simulink model "battery_system_CV_PID"  (R2022a)
settings: Solver=VariableStepAuto  StartTime=0.0  StopTime=10.0  RelTol=1e-3
model workspace (MAT data in the model file):
  AN.EqPotentialHandle = 'E_eqGraphite'
  AN.i_oHandle = 'i_oC6'
  AN.sigmaHandle = 'sigmaC6'
  AN.D_oHandle = 'D_o_Graphite'
  AN.k_o = 3.80589129595e-09
  AN.alpha_a = 0.5
  AN.alpha_c = 0.5
  AN.C_dl = 3e-06
  AN.R_SEI = 0.00733702042142
  AN.sigma = 100
  AN.D_o = 3e-13
  AN.MW = 72.0642
  AN.MW_Lith = 79.0052
  AN.specCap = 350
  AN.rho = 2266
  AN.c_p = 720
  AN.k = 0.6
  AN.C_Li_max = 28.4851292094
  AN.del_z = 0.316227766017
  AN.del_y = 0.316227766017
  AN.L = 0.0001
  AN.r_p = 1.25e-05
  AN.eps_ed = 0.320700992698
  AN.eps_b = 0.172
  AN.A_geo = 1
  AN.gamma_brug = 1
  AN.alpha_brug = 1.5
  AN.del_x = 1e-05
  AN.x_vec = [5e-06 1.5e-05 2.5e-05 3.5e-05 4.5e-05 5.5e-05 6.5e-05 7.5e-05 8.5e-05 9.5e-05]
  AN.x_half_vec = [0 1e-05 2e-05 3e-05 4e-05 5e-05 6e-05 7e-05 8e-05 9e-05 0.0001]
  AN.del_r = 1.25e-06
  AN.r_vec = [6.25e-07 1.875e-06 3.125e-06 4.375e-06 5.625e-06 6.875e-06 8.125e-06 9.375e-06 1.0625e-05 1.1875e-05]
  AN.r_half_vec = [0 1.25e-06 2.5e-06 3.75e-06 5e-06 6.25e-06 7.5e-06 8.75e-06 1e-05 1.125e-05 1.25e-05]
  AN.eps_el = 0.507299007302
  AN.A_c = 0.1
  AN.Vol = 1e-05
  AN.dVol = 1e-06
  AN.V_sphere = 8.18123086872e-15
  AN.V_ed = 3.20700992698e-06
  AN.V_el = 5.07299007302e-06
  AN.dVol_el = 5.07299007302e-07
  AN.Np_tot = 391996018.501
  AN.Np_CV = 39199601.8501
  AN.A_surf = 1.96349540849e-09
  AN.A_surf_tot = 0.769682382475
  AN.A_surf_CV = 0.0769682382475
  AN.A_s = 76968.2382475
  AN.dVol_r = [8.18123086872e-18; 5.72686160811e-17; 1.55443386506e-16; 3.02705542143e-16; 4.99055082992e-16; 7.44492009054e-16; 1.03901632033e-15; 1.38262801681e-15; 1.77532709851e-15; 2.21711356542e-15]
  AN.Cap = 2.44837153197
  C = [0 0 -0.999999993923 0 0 0 0 0 0 0 0 0 0 0 0 0 0 0 0 0 0 0 0 0 0 0 0 0 0 0 0 0 0 0 0 0 0 0 0 0 0 0 0 0 0 0 0 0 0 0 0 0 0 0 0 0 0 0 0 0 0 0 0 0 0 0 0 0 0 0 0 0 0 0 0 0 0 0 0 0 0 0 0 0 0 0 0 0 0 0 0 0 0 0 0 0 0 0 0 0 0 0 0 0 0 0 0 0 0 0 0 0 0 0 0 0 0 0 0 0 0 0 0 0 0 0 0 0 0 0 0 0 0 0 0 0 0 0 0 0 0 0 0 0 0 0 0 0 0 0 0 0 0 0 0 0 0 0 0 0 0 0 0 0 0 0 0 0 0 0 0 0 0 0 0 0 0 0 0 0 0 0 0 0 0 0 0 0 0 0 0 0 0 0 0 0 0 0 0 0 0 0 0 0 0 0 0 0 0 0 0 0 0 0 0 0 0 0 0 0 0 0 0 0 0 0 0 0 0 0 0 0 0 0 0 0 0 0 0 0 0 0 0 0 0 0 0 0 0 0 0 0 0 0 0 0 0 0 0 0 0 0 0 0 0 0 0 0 0 0 0 0 0 0 0 0 0 0 0 0 0 0 0 0 0 0 0 0 0 0 0 0 0 0 0 0 0 0 0 0 0 0 0 0 0 0 0 0 0 0 0 0 0 0 0 0 0 0 0 0 0 0 0 0 0 0 0 0 0 0 0 0 0 0 0 0 0 0 0 0 0.999999999995 0 0 0 0 0 0 0 0 0 0 0 0 0 0]
  CA.EqPotentialHandle = 'E_eqNMC'
  CA.i_oHandle = 'i_oC6'
  CA.sigmaHandle = 'sigmaNMC'
  CA.D_oHandle = 'D_o_NMC532'
  CA.k_o = 9.72997022034e-10
  CA.alpha_a = 0.5
  CA.alpha_c = 0.5
  CA.C_dl = 1e-06
  CA.R_SEI = 0.00611911635272
  CA.sigma = 3.8
  CA.D_o = 5e-13
  CA.MW = 89.61275
  CA.MW_Lith = 96.55375
  CA.specCap = 170
  CA.rho = 2739.6961
  CA.c_p = 720
  CA.k = 0.6
  CA.C_Li_max = 40.5441490868
  CA.del_z = 0.316227766017
  CA.del_y = 0.316227766017
  CA.L = 0.0001
  CA.r_p = 5e-06
  CA.eps_ed = 0.442994582877
  CA.eps_b = 0.259
  CA.A_geo = 1
  CA.gamma_brug = 1
  CA.alpha_brug = 1.5
  CA.del_x = 1e-05
  CA.x_vec = [0.000135 0.000145 0.000155 0.000165 0.000175 0.000185 0.000195 0.000205 0.000215 0.000225]
  CA.x_half_vec = [0.00013 0.00014 0.00015 0.00016 0.00017 0.00018 0.00019 0.0002 0.00021 0.00022 0.00023]
  CA.del_r = 5e-07
  CA.r_vec = [2.5e-07 7.5e-07 1.25e-06 1.75e-06 2.25e-06 2.75e-06 3.25e-06 3.75e-06 4.25e-06 4.75e-06]
  CA.r_half_vec = [0 5e-07 1e-06 1.5e-06 2e-06 2.5e-06 3e-06 3.5e-06 4e-06 4.5e-06 5e-06]
  CA.eps_el = 0.298005417123
  CA.A_c = 0.1
  CA.Vol = 1e-05
  CA.dVol = 1e-06
  CA.V_sphere = 5.23598775598e-16
  CA.V_ed = 4.42994582877e-06
  CA.V_el = 2.98005417123e-06
  CA.dVol_el = 2.98005417123e-07
  CA.Np_tot = 8460573315.33
  CA.Np_CV = 846057331.533
  CA.A_surf = 3.14159265359e-10
  CA.A_surf_tot = 2.65796749726
  CA.A_surf_CV = 0.265796749726
  CA.A_s = 265796.749726
  CA.dVol_r = [5.23598775598e-19; 3.66519142919e-18; 9.94837673637e-18; 1.93731546971e-17; 3.19395253115e-17; 4.76474885794e-17; 6.6497044501e-17; 8.84881930761e-17; 1.13620934305e-16; 1.41895268187e-16]
  CA.Cap = 4.81377102891
  CONS.F = 96485338.3
  CONS.R = 8314.472
  CONS.T = 298.15
  CV_ref = 3.74905480499
  EL.tf_numHandle = 'transferenceNumber'
  EL.ActivityHandle = 'activity'
  EL.D_o_Li_ionHandle = 'D_oLiion'
  EL.kappaHandle = 'kappa'
  EL.D_o_Li_ion = 7.5e-11
  EL.kappa = 0.28
  EL.C = 1
  EL.tf_num = 0.363
  EL.Activity = 1
  EL.rho = 2266
  EL.c_p = 720
  EL.k = 470
  EL.gamma_brug = 1
  EL.alpha_brug = 1.5
  FLAG.AN_LI_FOIL = 0
  FLAG.CA_LI_FOIL = 0
  FLAG.R_AN = 1
  FLAG.R_CA = 1
  FLAG.COE = 0
  FLAG.T_BC_AN = 4
  FLAG.T_BC_CA = 4
  FLAG.CV_CONV = 0
  FLAG.HEAT_GEN_TOTAL = 1
  FLAG.HEAT_GEN_IONIC = 1
  FLAG.HEAT_GEN_ELECTRIC = 1
  FLAG.HEAT_GEN_RXN = 1
  FLAG.HEAT_GEN_CHEM_RXN = 0
  FLAG.V_SEI = 1
  FLAG.SEI_growth = 0
  FLAG.HeatGen = 0
  FLAG.Bruggeman = 0
  FLAG.BRUG_ED = 1
  FLAG.BRUG_EL = 1
  FLAG.BRUG_sigma = 1
  FLAG.BRUG_kappa = 1
  FLAG.BRUG_activity = 0
  FLAG.BRUG_D_Liion = 1
  FLAG.BRUG_tf_num = 0
  FLAG.BRUG_D_o_AN = 0
  FLAG.BRUG_D_o_CA = 0
  FLAG.Newman_i_o = 1
  FLAG.preDefined_C_max = 1
  FLAG.CONSTANT_PROPS_FROM_HANDLES = 0
  FLAG.VARIABLE_PROPS_FROM_HANDLES = 0
  FLAG.VARIABLE_kappa = 1
  FLAG.VARIABLE_activity = 0
  FLAG.VARIABLE_D_Liion = 0
  FLAG.VARIABLE_tf_num = 0
  FLAG.VARIABLE_D_o_AN = 0
  FLAG.VARIABLE_D_o_CA = 0
  FLAG.SaveSolnDiscreteTime = 1
  FLAG.SaveSystemForEst = 0
  FLAG.doPostProcessing = 1
  FLAG.ReduceSolnTime = 0
  FLAG.Plot = 1
  FLAG.PRBS_predefinded = 0
  K_D = 0
  K_I = -7437.93380511
  K_P = 0
  K_algb = [0 0 0 0 0 0 0 0 0 0 0 0 ... (126025 elements, 355x355)]
  M_cross = [1 0 0 0 0 0 0 0 0 0 0 0 ... (126025 elements, 355x355)]
  N.N_CV_AN = 10
  N.N_CV_SEP = 5
  N.N_CV_CA = 10
  N.N_R_AN = 10
  N.N_R_CA = 10
  N.N_R_max = 10
  N.N_ES_var = 6
  N.N_SV_nR = 7
  N.N_SV_SEP = 3
  N.N_prop = 19
  N.N_SV_AN = 17
  N.N_SV_CA = 17
  N.N_SV_AN_tot = 170
  N.N_SV_SEP_tot = 15
  N.N_SV_CA_tot = 170
  N.N_SV_tot = 355
  N.N_CV_tot = 25
  N.CV_Region_AN = [1 2 3 4 5 6 7 8 9 10]
  N.CV_Region_SEP = [11 12 13 14 15]
  N.CV_Region_CA = [16 17 18 19 20 21 22 23 24 25]
  N.N_diff = 270
  N.N_algb = 85
  P.T = 1
  P.del_phi = 2
  P.phi_ed = 3
  P.V_1 = 4
  P.V_2 = 5
  P.i_PS = 6
  P.C_Liion = 7
  P.C_Li = 8
  P.C_Li_surf_AN = 17
  P.C_Li_surf_CA = 17
  P.C_Li_surf_max = 17
  P.SEP.T = 1
  P.SEP.phi_el = 2
  P.SEP.C_Liion = 3
  P.phi_el = 18
  P.ES.del_phi = 1
  P.ES.phi_ed = 2
  P.ES.V_1 = 3
  P.ES.V_2 = 4
  P.ES.i_PS = 5
  P.ES.i_dl = 6
  P.sigma = 1
  P.kappa = 2
  P.R_SEI = 3
  P.k = 4
  P.rho = 5
  P.c_p = 6
  P.D_o_Li_ion = 7
  P.activity = 8
  P.tf_num = 9
  P.D_o = 10
  PROPS = [100 0.28 0.00733702042142 0.6 2266 720 7.5e-11 1 0.363 3e-13 3e-13 3e-13 ... (475 elements, 19x25)]
  SEP.rho = 2266
  SEP.c_p = 720
  SEP.k = 0.6
  SEP.del_z = 0.316227766017
  SEP.del_y = 0.316227766017
  SEP.L = 3e-05
  SEP.eps = 1
  SEP.del_x = 6e-06
  SEP.x_vec = [0.000103 0.000109 0.000115 0.000121 0.000127]
  SEP.x_half_vec = [0.0001 0.000106 0.000112 0.000118 0.000124 0.00013]
  SEP.eps_el = 1
  SEP.A_c = 0.1
  SEP.Vol = 3e-06
  SEP.dVol = 6e-07
  SEP.V_el = 3e-06
  SEP.dVol_el = 6e-07
  SIM.results_filename = 'TestingSimulink_KPCont_1C20_CVTest_SOC50_SOC0.mat'
  SIM.SimMode = 4
  SIM.SOC_start = 0
  SIM.SaveTimeStep = 2
  SIM.DiscreteTimeStep = 0.001
  SIM.ZeroTime = 0.01
  SIM.cell_geo = 'p'
  SIM.Temp_start = 298.15
  SIM.T_inf = 298.15
  SIM.h = 1
  SIM.initial_offset = 0
  SIM.VoltageMax = 4.2
  SIM.VoltageMin = 3.4
  SIM.AnodeFormation_X = 0
  SIM.CathodeFormation_X = 1
  SIM.x_vec = [5e-06 1.5e-05 2.5e-05 3.5e-05 4.5e-05 5.5e-05 6.5e-05 7.5e-05 8.5e-05 9.5e-05 0.000103 0.000109 0.000115 0.000121 0.000127 0.000135 0.000145 0.000155 0.000165 0.000175 0.000185 0.000195 0.000205 0.000215 0.000225]
  SIM.x_half_vec = [0 1e-05 2e-05 3e-05 4e-05 5e-05 6e-05 7e-05 8e-05 9e-05 0.0001 0.000106 0.000112 0.000118 0.000124 0.00013 0.00014 0.00015 0.00016 0.00017 0.00018 0.00019 0.0002 0.00021 0.00022 0.00023]
  SIM.CV_vec = [1e-06 1e-06 1e-06 1e-06 1e-06 1e-06 1e-06 1e-06 1e-06 1e-06 6e-07 6e-07 6e-07 6e-07 6e-07 1e-06 1e-06 1e-06 1e-06 1e-06 1e-06 1e-06 1e-06 1e-06 1e-06]
  SIM.A_surf_CV_vec = [0.0769682382475 0.0769682382475 0.0769682382475 0.0769682382475 0.0769682382475 0.0769682382475 0.0769682382475 0.0769682382475 0.0769682382475 0.0769682382475 0 0 0 0 0 0.265796749726 0.265796749726 0.265796749726 0.265796749726 0.265796749726 0.265796749726 0.265796749726 0.265796749726 0.265796749726 0.265796749726]
  SIM.x_ini = 0.0592
  SIM.y_ini = 0.831089802855
  SIM.A_c = 0.1
  SIM.Cell_Cap = 2.44837153197
  SIM.current_MO_step = 2
  SIM.phi_guess = [0.272411056579; 0; -0.272411056579; -0.272411056579; 0; 0; 0.272411056579; 0; -0.272411056579; -0.272411056579; 0; 0; 0.272411056579; 0; -0.272411056579; -0.272411056579; 0; 0; 0.272411056579; 0; -0.272411056579; -0.272411056579; 0; 0; 0.272411056579; 0; -0.272411056579; -0.272411056579; 0; 0; 0.272411056579; 0; -0.272411056579; -0.272411056579; 0; 0; 0.272411056579; 0; -0.272411056579; -0.272411056579; 0; 0; 0.272411056579; 0; -0.272411056579; -0.272411056579; 0; 0; 0.272411056579; 0; -0.272411056579; -0.272411056579; 0; 0; 0.272411056579; 0; -0.272411056579; -0.272411056579; 0; 0; -0.272411056579; -0.272411056579; -0.272411056579; -0.272411056579; -0.272411056579; 3.70383165012; 3.43142059355; -0.272411056579; -0.272411056579; 0; 0; 3.70383165012; 3.43142059355; -0.272411056579; -0.272411056579; 0; 0; 3.70383165012; 3.43142059355; -0.272411056579; -0.272411056579; 0; 0; 3.70383165012; 3.43142059355; -0.272411056579; -0.272411056579; 0; 0; 3.70383165012; 3.43142059355; -0.272411056579; -0.272411056579; 0; 0; 3.70383165012; 3.43142059355; -0.272411056579; -0.272411056579; 0; 0; 3.70383165012; 3.43142059355; -0.272411056579; -0.272411056579; 0; 0; 3.70383165012; 3.43142059355; -0.272411056579; -0.272411056579; 0; 0; 3.70383165012; 3.43142059355; -0.272411056579; -0.272411056579; 0; 0; 3.70383165012; 3.43142059355; -0.272411056579; -0.272411056579; 0; 0; -1.22418576599]
  SIM.SV_IC = [298.15 0.272411056579 -1.43578558837e-26 -0.272411056579 -0.272411056579 -1.22824256273e-29 1 1.6863196492 1.6863196492 1.6863196492 1.6863196492 1.6863196492 ... (355 elements, 355x1)]
  SIM.M = [1 0 0 0 0 0 0 0 0 0 0 0 ... (126025 elements, 355x355)]
  SIM.diff_idx = [1 2 7 8 9 10 11 12 13 14 15 16 17 18 19 24 25 26 27 28 29 30 31 32 33 34 35 36 41 42 43 44 45 46 47 48 49 50 51 52 53 58 59 60 61 62 63 64 65 66 67 68 69 70 75 76 77 78 79 80 81 82 83 84 85 86 87 92 93 94 95 96 97 98 99 100 101 102 103 104 109 110 111 112 113 114 115 116 117 118 119 120 121 126 127 128 129 130 131 132 133 134 135 136 137 138 143 144 145 146 147 148 149 150 151 152 153 154 155 160 161 162 163 164 165 166 167 168 169 170 171 173 174 176 177 179 180 182 183 185 186 187 192 193 194 195 196 197 198 199 200 201 202 203 204 209 210 211 212 213 214 215 216 217 218 219 220 221 226 227 228 229 230 231 232 233 234 235 236 237 238 243 244 245 246 247 248 249 250 251 252 253 254 255 260 261 262 263 264 265 266 267 268 269 270 271 272 277 278 279 280 281 282 283 284 285 286 287 288 289 294 295 296 297 298 299 300 301 302 303 304 305 306 311 312 313 314 315 316 317 318 319 320 321 322 323 328 329 330 331 332 333 334 335 336 337 338 339 340 345 346 347 348 349 350 351 352 353 354 355]
  SIM.algb_idx = [3 4 5 6 20 21 22 23 37 38 39 40 54 55 56 57 71 72 73 74 88 89 90 91 105 106 107 108 122 123 124 125 139 140 141 142 156 157 158 159 172 175 178 181 184 188 189 190 191 205 206 207 208 222 223 224 225 239 240 241 242 256 257 258 259 273 274 275 276 290 291 292 293 307 308 309 310 324 325 326 327 341 342 343 344]
  SV_IC = [298.15 0.0999631520085 0 -0.101224623555 -0.102074642283 -0.171932402214 0.987757586119 14.5346948901 14.535438374 14.5369252829 14.5391554953 14.5421288288 ... (355 elements, 355x1)]
  SampTime = 2
  U_NV_NT = [0 0 0 0 0 0 0 0 0 0 0 0 ... (126025 elements, 355x355)]
  i_user_IC = -1.22418576599
values from neighbouring files (symbols this model uses):
  SIM = rmfield(SIM,'fsolve_options')    [runCC.m]    (also in runCVHold.m = rmfield(SIM,'Controller_MO_File'))
(part 1 of 2)
settings Model: Creator=tyevans  LastModifiedBy=tyevans
settings DataIOCC: OutputTimes=1:1:5000

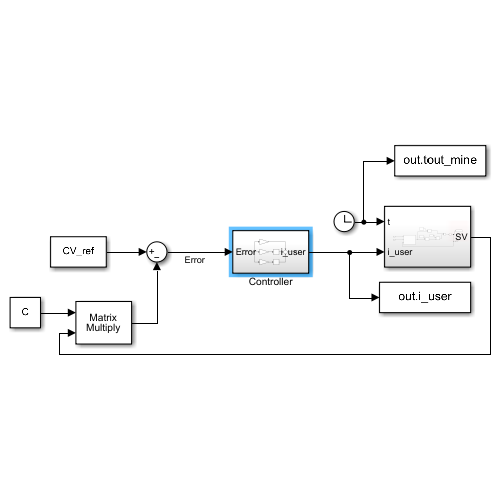
[thumbnail: Simulink's stored preview of the top-level diagram]
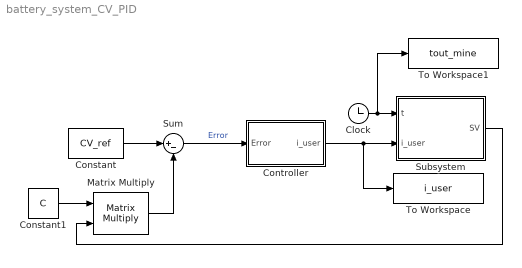
== system battery_system_CV_PID ==
  Clock : Clock
  Constant : Constant  Value=CV_ref  VectorParams1D=off
  Constant1 : Constant  Value=C  VectorParams1D=off
  Controller : Subsystem
  Matrix Multiply : Product  Multiplication=Matrix(*)
  Subsystem : Subsystem
  Sum : Sum  Inputs=|+-
  To Workspace : ToWorkspace  VariableName=i_user  SampleTime=SampTime
      settings: Save2DSignal=2-D array (concatenate along first dimension)
  To Workspace1 : ToWorkspace  VariableName=tout_mine  SampleTime=SampTime
      settings: Save2DSignal=2-D array (concatenate along first dimension)
  wires:
  Clock/1 -> To Workspace1/1, Subsystem/1(t)
  Constant/1 -> Sum/1
  Constant1/1 -> Matrix Multiply/1
  Matrix Multiply/1 -> Sum/2
  Subsystem/1(SV) -> Matrix Multiply/2
  Controller/1(i_user) -> To Workspace/1, Subsystem/2(i_user)
  Sum/1 -> Controller/1(Error)  "Error"
